simulink model "Sim_01"  (R2024b)
settings: Solver=VariableStepAuto  StartTime=0.0  StopTime=timeOfSimulation  RelTol=1e-3
undefined symbols (not defined in the file): C, H, K_m, K_r, tau_m, tau_r
settings Model: Creator=diegoalfonsocosta  LastModifiedBy=diegoalfonsocosta

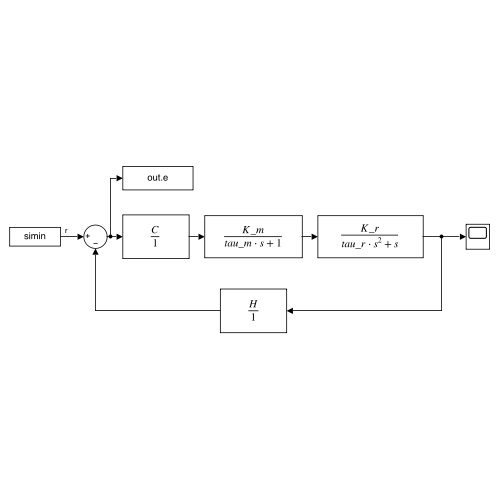
[thumbnail: Simulink's stored preview of the top-level diagram]
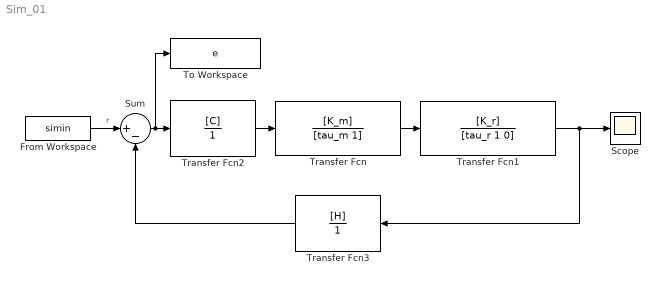
== system Sim_01 ==
  From Workspace : FromWorkspace  VariableName=simin
  Scope : Scope
  Sum : Sum  Inputs=|+-
  To Workspace : ToWorkspace  VariableName=e  SaveFormat=Timeseries  SampleTime=-1
  Transfer Fcn : TransferFcn  Numerator=[K_m]  Denominator=[tau_m 1]
  Transfer Fcn1 : TransferFcn  Numerator=[K_r]  Denominator=[tau_r 1 0]
  Transfer Fcn2 : TransferFcn  Numerator=[C]  Denominator=[1]
  Transfer Fcn3 : TransferFcn  Numerator=[H]  Denominator=[1]
  wires:
  Transfer Fcn/1 -> Transfer Fcn1/1
  Transfer Fcn1/1 -> Scope/1, Transfer Fcn3/1
  Transfer Fcn2/1 -> Transfer Fcn/1
  Sum/1 -> To Workspace/1, Transfer Fcn2/1
  From Workspace/1 -> Sum/1  "r"
  Transfer Fcn3/1 -> Sum/2
